simulink model "R_V_OprnLoop"  (R2020a)
settings: Solver=ode4  StartTime=0.0  StopTime=20  FixedStep=0.001  RelTol=1e-3
InitFcn:
  | m = 1   ; % ball weight (kg)
  | d = 0.05; % gear rediuce (m)
  | a = 0.02; % ball rediuce (m)
  | L = 1   ; % bar length (m)
  | g = 9.8 ; % m/s^2
settings Model: Creator=Ali  LastModifiedBy=Ali

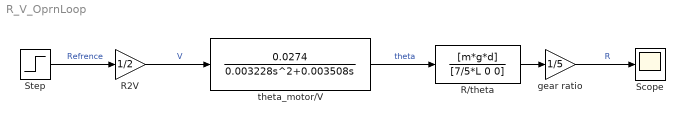
== system R_V_OprnLoop ==
  R/theta : TransferFcn  Numerator=[m*g*d]  Denominator=[7/5*L 0 0]
  R2V : Gain  Gain=1/2
  Scope : Scope
  Step : Step  Time=0  After=0.5  SampleTime=0
  gear ratio : Gain  Gain=1/5
  theta_motor/V : TransferFcn  Numerator=[0.0274]  Denominator=[0.003228 0.003508 0]
  wires:
  R/theta/1 -> gear ratio/1
  Step/1 -> R2V/1  "Refrence"
  theta_motor/V/1 -> R/theta/1  "theta"
  gear ratio/1 -> Scope/1  "R"
  R2V/1 -> theta_motor/V/1  "V"
